simulink model "mainSimulink_localPi_IMU"  (R2021a)
settings: Solver=VariableStepAuto  StartTime=0.0  StopTime=inf  FixedStep=samplingTime  RelTol=1e-3
model workspace (MATLAB code in the model file):
  | %% Simulink settings
  | controllerFile = 'directFFcontroller';
  | set_param('mainSimulink_localPi_IMU/Subsystem Reference', 'ReferencedSubsystem', controllerFile);
  | %% Display settings
  | scopeTimeSpan = 30;
  | 
  | %% Robot settings (must match Python)
  | sensorFreq = 125;
  | actuatorFreq = 250;
  | TCPport = 12345;
  | dataSize = 4;
  | sensorSamplingTime = 1/sensorFreq;
  | actuatorTime = 1/actuatorFreq;
undefined symbols (not defined in the file): f
libraries: instrumentlib x2
settings Model: Creator=chukh  LastModifiedBy=chukh

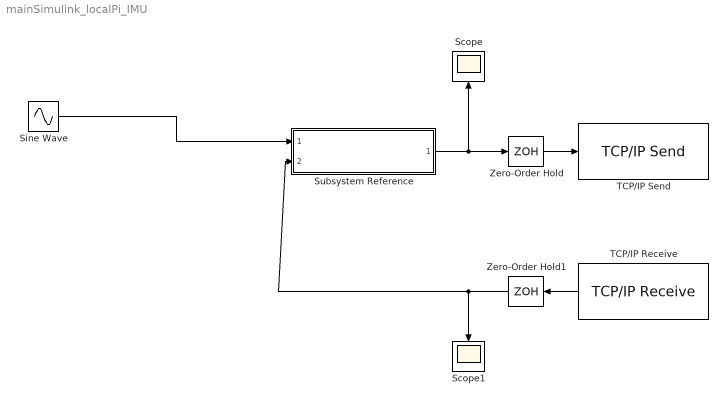
== system mainSimulink_localPi_IMU ==
  Scope : Scope
  Scope1 : Scope
  Sine Wave : Sin  Amplitude=0.5  Bias=0.5  SampleTime=0
  Subsystem Reference : Subsystem  ReferencedSubsystem=directFFcontroller
  TCP/IP Receive : instrumentlib/TCP//IP Receive  Host=server.softrobot  Port=TCPport  DataSize=dataSize  EnableBlockingMode=on  Timeout=0.5  SampleTime=sensorSamplingTime  DataType=double  ByteOrder=LittleEndian  ASCIIFormatting=%f,  Terminator=LF
  TCP/IP Send : instrumentlib/TCP//IP Send  Host=server.softrobot  Port=TCPport  EnableBlockingMode=on  Timeout=0.5  ByteOrder=LittleEndian  TransferDelay=on
  Zero-Order Hold : ZeroOrderHold  SampleTime=actuatorTime
  Zero-Order Hold1 : ZeroOrderHold  SampleTime=actuatorTime
  wires:
  Subsystem Reference/1 -> Zero-Order Hold/1, Scope/1
  TCP/IP Receive/1 -> Zero-Order Hold1/1
  Zero-Order Hold/1 -> TCP/IP Send/1
  Zero-Order Hold1/1 -> Scope1/1, Subsystem Reference/2
  Sine Wave/1 -> Subsystem Reference/1
